simulink model "testGaitGeneration"  (R2016b)
settings: Solver=FixedStepAuto  StartTime=0.0  StopTime=12  FixedStep=0.001  RelTol=1e-3
undefined symbols (not defined in the file): angleHip, angleKnee, GaitGenerator, lookUpTable, stateMachineHandler
settings Model: DataDictionary=ModelDictionary.sldd  Creator=Taeke  LastModifiedBy=Taeke

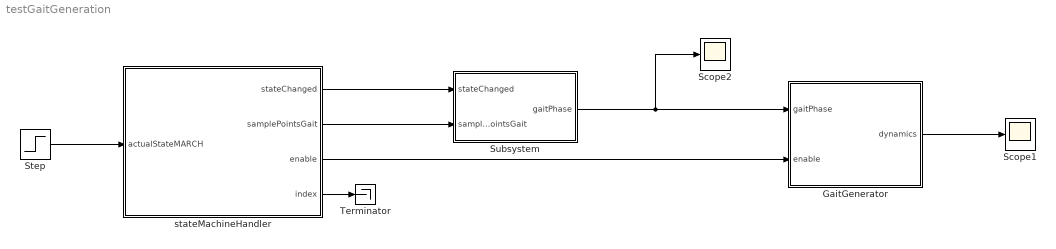
== system testGaitGeneration ==
  GaitGenerator : Subsystem  AncestorBlock=lookUpTable/GaitGenerator
  Scope1 : Scope
  Scope2 : Scope
  Step : Step  Time=5  SampleTime=0
  Subsystem : Subsystem  AncestorBlock=determinePhase/stateMachineHandler/Subsystem
  Terminator : Terminator
  stateMachineHandler : Subsystem  AncestorBlock=stateMachineHandler/stateMachineHandler
  wires:
  stateMachineHandler/1(stateChanged) -> Subsystem/1(stateChanged)
  stateMachineHandler/3(enable) -> GaitGenerator/2(enable)
  Step/1 -> stateMachineHandler/1(actualStateMARCH)
  Subsystem/1(gaitPhase) -> Scope2/1, GaitGenerator/1(gaitPhase)
  stateMachineHandler/2(samplePointsGait) -> Subsystem/2(samplePointsGait)
  stateMachineHandler/4(index) -> Terminator/1
  GaitGenerator/1(dynamics) -> Scope1/1

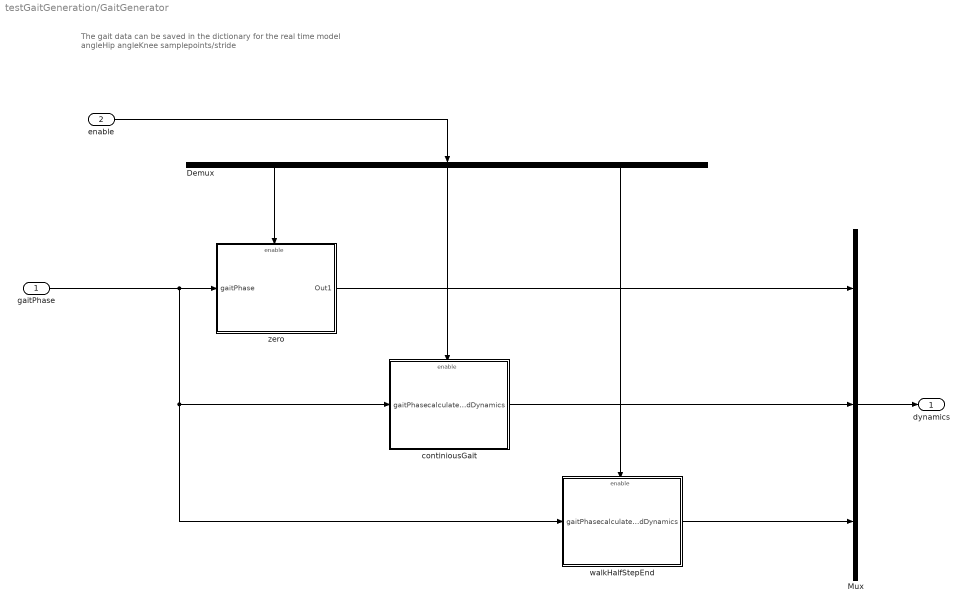
== system testGaitGeneration/GaitGenerator ==
  note: The gait data can be saved in the dictionary for the real time model
      | angleHip
      | angleKnee
      | samplepoints/stride
  gaitPhase : Inport
  enable : Inport  Port=2
  Demux : Demux  Outputs=3
  Mux : Mux  Inputs=3
  continiousGait : Subsystem
  walkHalfStepEnd : Subsystem
  zero : Subsystem
  dynamics : Outport
  wires:
  Demux/1 -> zero/Enable
  Demux/2 -> continiousGait/Enable
  Demux/3 -> walkHalfStepEnd/Enable
  gaitPhase/1 -> walkHalfStepEnd/1(gaitPhase), continiousGait/1(gaitPhase), zero/1(gaitPhase)
  continiousGait/1(calculatedDynamics) -> Mux/2
  enable/1 -> Demux/1
  Mux/1 -> dynamics/1
  walkHalfStepEnd/1(calculatedDynamics) -> Mux/3
  zero/1(Out1) -> Mux/1

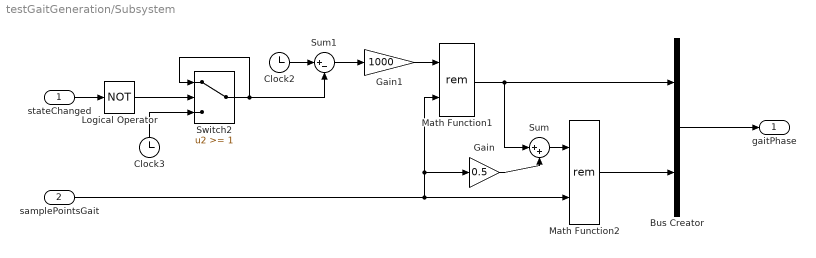
== system testGaitGeneration/Subsystem ==
  stateChanged : Inport
  samplePointsGait : Inport  Port=2
  Bus Creator : BusCreator  Inputs=2
  Clock2 : Clock
  Clock3 : Clock
      settings: Decimation=4
  Gain : Gain  Gain=0.5
  Gain1 : Gain  Gain=1000
  Logical Operator : Logic  Operator=NOT  AllPortsSameDT=off  OutDataTypeStr=boolean
  Math Function1 : Math  Operator=rem  SaturateOnIntegerOverflow=on
  Math Function2 : Math  Operator=rem  SaturateOnIntegerOverflow=on
  Sum : Sum  Inputs=|++
  Sum1 : Sum  Inputs=|+-  SaturateOnIntegerOverflow=on  InputSameDT=on  OutDataTypeStr=Inherit: Same as first input
  Switch2 : Switch  Threshold=1  RndMeth=Zero
  gaitPhase : Outport
  wires:
  Gain1/1 -> Math Function1/1
  Sum1/1 -> Gain1/1
  Clock2/1 -> Sum1/1
  Clock3/1 -> Switch2/3
  Switch2/1 -> Switch2/1, Sum1/2
  Logical Operator/1 -> Switch2/2
  stateChanged/1 -> Logical Operator/1
  samplePointsGait/1 -> Gain/1, Math Function1/2, Math Function2/2
  Math Function1/1 -> Sum/1, Bus Creator/1
  Gain/1 -> Sum/2
  Sum/1 -> Math Function2/1
  Math Function2/1 -> Bus Creator/2
  Bus Creator/1 -> gaitPhase/1

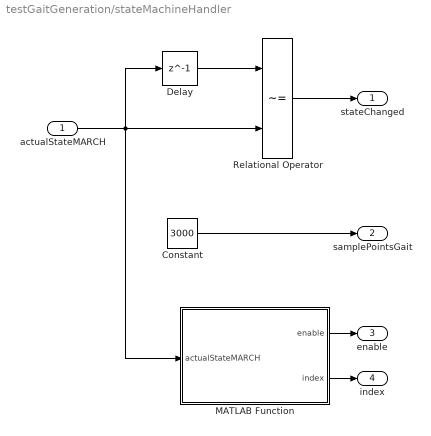
== system testGaitGeneration/stateMachineHandler ==
  actualStateMARCH : Inport
  Constant : Constant  Value=3000
  Delay : Delay  DelayLength=1  InitialCondition=0
  MATLAB Function : MATLAB Function  TreatAsAtomicUnit=on
  Relational Operator : RelationalOperator  Operator=~=  OutDataTypeStr=boolean  RndMeth=Simplest
  stateChanged : Outport  BusOutputAsStruct=on
  samplePointsGait : Outport  Port=2
  enable : Outport  Port=3
  index : Outport  Port=4
  wires:
  Relational Operator/1 -> stateChanged/1
  Delay/1 -> Relational Operator/1
  actualStateMARCH/1 -> MATLAB Function/1(actualStateMARCH), Relational Operator/2, Delay/1
  Constant/1 -> samplePointsGait/1
  MATLAB Function/1(enable) -> enable/1
  MATLAB Function/2(index) -> index/1

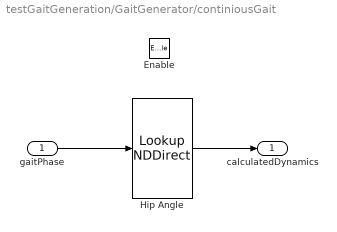
== system testGaitGeneration/GaitGenerator/continiousGait ==
  gaitPhase : Inport
  Enable : EnablePort
  Hip Angle : LookupNDDirect  NumberOfTableDimensions=1  Table=angleHip
  calculatedDynamics : Outport  BusOutputAsStruct=on
  wires:
  gaitPhase/1 -> Hip Angle/1
  Hip Angle/1 -> calculatedDynamics/1

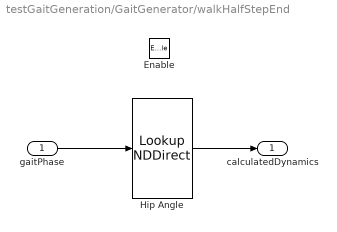
== system testGaitGeneration/GaitGenerator/walkHalfStepEnd ==
  gaitPhase : Inport
  Enable : EnablePort
  Hip Angle : LookupNDDirect  NumberOfTableDimensions=1  Table=angleHip
  calculatedDynamics : Outport  BusOutputAsStruct=on
  wires:
  gaitPhase/1 -> Hip Angle/1
  Hip Angle/1 -> calculatedDynamics/1

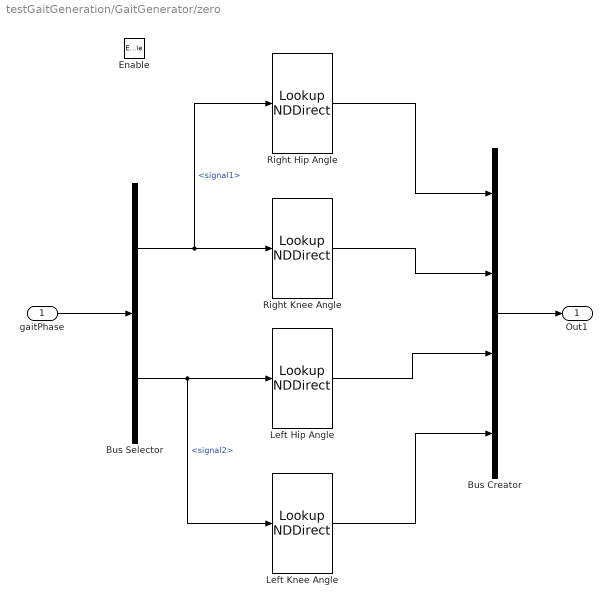
== system testGaitGeneration/GaitGenerator/zero ==
  gaitPhase : Inport
  Enable : EnablePort
  Bus Creator : BusCreator  Inputs=4  OutDataTypeStr=Bus: calculatedAngles
  Bus Selector : BusSelector  OutputSignals=signal1,signal2
  Left Hip Angle : LookupNDDirect  NumberOfTableDimensions=1  Table=angleHip
  Left Knee Angle : LookupNDDirect  NumberOfTableDimensions=1  Table=angleKnee
  Right Hip Angle : LookupNDDirect  NumberOfTableDimensions=1  Table=angleHip
  Right Knee Angle : LookupNDDirect  NumberOfTableDimensions=1  Table=angleKnee
  Out1 : Outport
  wires:
  Right Hip Angle/1 -> Bus Creator/1
  gaitPhase/1 -> Bus Selector/1
  Bus Selector/1 -> Right Hip Angle/1, Right Knee Angle/1  "<signal1>"
  Bus Selector/2 -> Left Knee Angle/1, Left Hip Angle/1  "<signal2>"
  Right Knee Angle/1 -> Bus Creator/2
  Left Hip Angle/1 -> Bus Creator/3
  Left Knee Angle/1 -> Bus Creator/4
  Bus Creator/1 -> Out1/1

== matlab function testGaitGeneration/stateMachineHandler/MATLAB Function ==
  data: enable output; actualStateMARCH input; index output
function [enable, index]= gaitSwitcher(actualStateMARCH)
%#codegen

% This function is supposed to take a state and switch between controllers.
% Currently it directly routes the input argument as the index. In the
% future this can be something different so I have left it open for
% future modifications.

% The u vector represents the controllers. When the vector consists out of
% zeros it will not enable any controller. In the case that an index is set
% to a non zero value, the controller which belongs to that index will be
% enabled.
u = zeros(3,1);

if actualStateMARCH
    u(actualStateMARCH) = 1;
end

index = actualStateMARCH;
enable = u;
